simulink model "truckt_ROS_mpc_8dof_2020a"  (R2020a)
settings: Solver=FixedStepAuto  StartTime=0.0  StopTime=40  FixedStep=0.001  RelTol=1e-3
model workspace (MAT data in the model file):
  Logfile_Data_Object = robotics.ros.BagSelection
  Logfile_Data_Object.FilePath = 'D:\robotruck_school\robotruck_school\ws\2025-05-22-09-01-20-filter.bag'
  Logfile_Data_Object.StartTime = 1747875680.55
  Logfile_Data_Object.EndTime = 1747876785.76
  Logfile_Data_Object.NumMessages = 154547
  Logfile_Data_Object.AvailableTopics = table
  Logfile_Data_Object.AvailableTopics.data{1} = [32976; 55257; 12; 11050; 55252]
  Logfile_Data_Object.AvailableTopics.data{2} = categorical
  Logfile_Data_Object.AvailableTopics.data{2}.categoryNames = {'robominer_msgs/ControlCmd'; 'robominer_msgs/GlobalPlan'; 'robominer_msgs/LocalPlan'; 'robominer_msgs/LocalizationData'; 'robominer_msgs/VcuData'}
  Logfile_Data_Object.AvailableTopics.data{2}.codes = [1; 4; 2; 3; 5]
  Logfile_Data_Object.AvailableTopics.data{3}{1} = '  uint32 Seq
    |   Time Stamp
    |   char FrameId
    | robominer_msgs/DriveMode TargetDriveMode
    |   uint8 Mode
    |   uint8 MANU
    |   uint8 TELE
    |   uint8 AUTO
    |   uint8 JOYTELE
    | robominer_msgs/Gear TargetGear
    |   uint8 Gear
    |   uint8 P
    |   uint8 R
    |   uint8 N
    |   uint8 D
    |   uint8 ShiftError
    | robominer_msgs/GearData TargetGearData
    |   uint8 GearData
    |   uint8 DEFAULT
    |   uint8 N
    |   uint8 D1
    |   uint8 D2
    |   uint8 D3
    |   uint8 D4
    |   uint8 D5
    |   uint8 D6
    |   uint8 D7
    |   uint8 R
    |   uint8 R1
    |   uint8 R2
    |   uint8 DOWN
    |   uint8 UP
    |   uint8 ShiftError
    | double TargetThrottle
    | double TargetBrake
    | double TargetSteering
    | '
  Logfile_Data_Object.AvailableTopics.data{3}{2} = '  uint32 Seq
    |   Time Stamp
    |   char FrameId
    | logical IsValid
    | double Latitude
    | double Longitude
    | double Altitude
    | double X
    | double Y
    | double Z
    | double Speed
    | double Vx
    | double Vy
    | double Vz
    | double Ax
    | double Ay
    | double Az
    | double Roll
    | double Pitch
    | double Yaw
    | double Wx
    | double Wy
    | double Wz
    | uint8 Solnsvs
    | uint8 Solnsvs2
    | uint8 Age
    | uint8 GgaAge
    | robominer_msgs/LocalizationStatus RtkStatus
    |   uint8 Status
    |   uint8 RTKINIT
    |   uint8 APOSIT
    |   uint8 RTCMDIFF
    |   uint8 NOTUSED
    |   uint8 RTKFIX
    |   uint8 RTKFLO
    |   uint8 RTKOTHER
    |   uint8 DATATIMOUT
    | '
  Logfile_Data_Object.AvailableTopics.data{3}{3} = '  uint32 Seq
    |   Time Stamp
    |   char FrameId
    | robominer_msgs/Waypoints Waypoints
    |   robominer_msgs/Waypoint[] Points
    |     double X
    |     double Y
    |     double Z
    |     double Latitude
    |     double Longitude
    |     double Altitude
    |     double Yaw
    |     double Pitch
    |     double Speed
    |     double Steering
    |     double Fs
    |     double Kappa
    |     double SpeedLimit
    |     robominer_msgs/Gear Gear
    |       uint8 Gear
    |       uint8 P
    |       uint8 R
    |       uint8 N
    |       uint8 D
    |       uint8 ShiftError
    |     robominer_msgs/GearData GearData
    |       uint8 GearData
    |       uint8 DEFAULT
    |       uint8 N
    |       uint8 D1
    |       uint8 D2
    |       uint8 D3
    |       uint8 D4
    |       uint8 D5
    |       uint8 D6
    |       uint8 D7
    |       uint8 R
    |       uint8 R1
    |       uint8 R2
    |       uint8 DOWN
    |       uint8 UP
    |       uint8 ShiftError
    |     robominer_msgs/WaypointType WaypointType
    |       uint8 PointType
    |       uint8 NORMAL
    |       uint8 LOAD
    |       uint8 DUMP
    |       uint8 WAIT
    |       uint8 AVOID
    |       uint8 REGION
    |     uint32 Index
    | '
  Logfile_Data_Object.AvailableTopics.data{3}{4} = '  uint32 Seq
    |   Time Stamp
    |   char FrameId
    | robominer_msgs/TaskType TaskType
    |   uint32 Type
    |   uint32 NORMAL
    |   uint32 LOAD
    |   uint32 DUMP
    |   uint32 PARKING
    |   uint32 BATTERYSWAP
    |   uint32 OTHERTASKS
    | robominer_msgs/Waypoints Waypoints
    |   robominer_msgs/Waypoint[] Points
    |     double X
    |     double Y
    |     double Z
    |     double Latitude
    |     double Longitude
    |     double Altitude
    |     double Yaw
    |     double Pitch
    |     double Speed
    |     double Steering
    |     double Fs
    |     double Kappa
    |     double SpeedLimit
    |     robominer_msgs/Gear Gear
    |       uint8 Gear
    |       uint8 P
    |       uint8 R
    |       uint8 N
    |       uint8 D
    |       uint8 ShiftError
    |     robominer_msgs/GearData GearData
    |       uint8 GearData
    |       uint8 DEFAULT
    |       uint8 N
    |       uint8 D1
    |       uint8 D2
    |       uint8 D3
    |       uint8 D4
    |       uint8 D5
    |       uint8 D6
    |       uint8 D7
    |       uint8 R
    |       uint8 R1
    |       uint8 R2
    |       uint8 DOWN
    |       uint8 UP
    |       uint8 ShiftError
    |     robominer_msgs/WaypointType WaypointType
    |       uint8 PointType
    |       uint8 NORMAL
    |       uint8 LOAD
    |       uint8 DUMP
    |       uint8 WAIT
    |       uint8 AVOID
    |       uint8 REGION
    |     uint32 Index
    | robominer_msgs/PlanningStatus Status
    |   uint8 Status
    |   char Msg
    |   uint8 IDLE
    |   uint8 PAUSED
    |   uint8 RUNNING
    |   uint8 DONE
    |   uint8 FAIL
    |   uint8 PAUSING
    |   uint8 STOPING
    |   uint8 OBSTACLE
    |   uint8 CUSP
    |   uint8 PLANNING
    |   uint8 STOPYIELD
    |   uint8 PASSYIELD
    | int32 NearestPointIndex
    | double Fs
    | double Fd
    | double TotalFs
    | int32 ValidPointNum
    | double RefYaw
    | double YawDeviation
    | '
  Logfile_Data_Object.AvailableTopics.data{3}{5} : char (value not decoded)
  Logfile_Data_Object.AvailableTopics.ndims = 2
  Logfile_Data_Object.AvailableTopics.nrows = 5
  Logfile_Data_Object.AvailableTopics.rownames = {'/guardian/control_cmd'; '/localization/localization_data'; '/planner/global_path'; '/planner/local_path'; '/vcu/vcu_data'}
  Logfile_Data_Object.AvailableTopics.nvars = 3
  Logfile_Data_Object.AvailableTopics.varnames = {'NumMessages', 'MessageType', 'MessageDefinition'}
  Logfile_Data_Object.AvailableTopics.props.useVariableNamesOriginal = 0
  Logfile_Data_Object.AvailableTopics.props.useDimensionNamesOriginal = 0
  Logfile_Data_Object.AvailableTopics.props.CustomProps = struct()
  Logfile_Data_Object.AvailableTopics.props.VariableCustomProps = struct()
  Logfile_Data_Object.AvailableTopics.props.versionSavedFrom = 4
  Logfile_Data_Object.AvailableTopics.props.minCompatibleVersion = 1
  Logfile_Data_Object.AvailableTopics.props.incompatibilityMsg = ''
  Logfile_Data_Object.AvailableTopics.props.VersionSavedFrom = 4
  Logfile_Data_Object.AvailableTopics.props.Description = ''
  Logfile_Data_Object.AvailableTopics.props.VariableNamesOriginal = {}
  Logfile_Data_Object.AvailableTopics.props.DimensionNames = {'Row', 'Variables'}
  Logfile_Data_Object.AvailableTopics.props.DimensionNamesOriginal = {}
  Logfile_Data_Object.AvailableTopics.props.UserData = []
  Logfile_Data_Object.AvailableTopics.props.VariableDescriptions = {}
  Logfile_Data_Object.AvailableTopics.props.VariableUnits = {}
  Logfile_Data_Object.AvailableTopics.props.VariableContinuity = {}
  Logfile_Data_Object.MessageList = table
  Logfile_Data_Object.MessageList.data{1} = [1747875680.55 1747875680.56 1747875680.57 1747875680.59 1747875680.6 1747875680.61 1747875680.63 1747875680.63 1747875680.65 1747875680.66 1747875680.67 1747875680.69 ... (154547 elements, 154547x1)]
  Logfile_Data_Object.MessageList.data{2} = categorical
  Logfile_Data_Object.MessageList.data{2}.categoryNames = {'/guardian/control_cmd'; '/localization/localization_data'; '/planner/global_path'; '/planner/local_path'; '/vcu/vcu_data'}
  Logfile_Data_Object.MessageList.data{2}.codes = [2 1 2 2 1 2 2 1 2 1 2 2 ... (154547 elements, 154547x1)]
  Logfile_Data_Object.MessageList.data{3} = categorical
  Logfile_Data_Object.MessageList.data{3}.categoryNames = {'robominer_msgs/ControlCmd'; 'robominer_msgs/LocalizationData'; 'robominer_msgs/GlobalPlan'; 'robominer_msgs/LocalPlan'; 'robominer_msgs/VcuData'}
  Logfile_Data_Object.MessageList.data{3}.codes = [2 1 2 2 1 2 2 1 2 1 2 2 ... (154547 elements, 154547x1)]
  Logfile_Data_Object.MessageList.data{4} = [6172 8389 8478 8703 8928 9017 9242 9467 9556 9781 9870 10095 ... (154547 elements, 154547x1)]
  Logfile_Data_Object.MessageList.ndims = 2
  Logfile_Data_Object.MessageList.nrows = 154547
  Logfile_Data_Object.MessageList.nvars = 4
  Logfile_Data_Object.MessageList.varnames = {'Time', 'Topic', 'MessageType', 'FileOffset'}
  Logfile_Data_Object.MessageList.props.useVariableNamesOriginal = 0
  Logfile_Data_Object.MessageList.props.useDimensionNamesOriginal = 0
  Logfile_Data_Object.MessageList.props.CustomProps = struct()
  Logfile_Data_Object.MessageList.props.VariableCustomProps = struct()
  Logfile_Data_Object.MessageList.props.versionSavedFrom = 4
  Logfile_Data_Object.MessageList.props.minCompatibleVersion = 1
  Logfile_Data_Object.MessageList.props.incompatibilityMsg = ''
  Logfile_Data_Object.MessageList.props.VersionSavedFrom = 4
  Logfile_Data_Object.MessageList.props.Description = ''
  Logfile_Data_Object.MessageList.props.VariableNamesOriginal = {}
  Logfile_Data_Object.MessageList.props.DimensionNames = {'Row', 'Variables'}
  Logfile_Data_Object.MessageList.props.DimensionNamesOriginal = {}
  Logfile_Data_Object.MessageList.props.UserData = []
  Logfile_Data_Object.MessageList.props.VariableDescriptions = {}
  Logfile_Data_Object.MessageList.props.VariableUnits = {}
  Logfile_Data_Object.MessageList.props.VariableContinuity = {}
  Logfile_Data_Object.TopicTypeMap = containers.Map
  Logfile_Data_Object.TopicTypeMap.serialization.keys = {'/guardian/control_cmd', '/localization/localization_data', '/planner/global_path', '/planner/local_path', '/vcu/vcu_data'}
  Logfile_Data_Object.TopicTypeMap.serialization.values = {'robominer_msgs/ControlCmd', 'robominer_msgs/LocalizationData', 'robominer_msgs/GlobalPlan', 'robominer_msgs/LocalPlan', 'robominer_msgs/VcuData'}
  Logfile_Data_Object.TopicTypeMap.serialization.uniformity = 1
  Logfile_Data_Object.TopicTypeMap.serialization.keyType = 'char'
  Logfile_Data_Object.TopicTypeMap.serialization.valueType = 'char'
  Logfile_Data_Object.TopicDefinitionMap = containers.Map
  Logfile_Data_Object.TopicDefinitionMap.serialization.keys = {'/guardian/control_cmd', '/localization/localization_data', '/planner/global_path', '/planner/local_path', '/vcu/vcu_data'}
  Logfile_Data_Object.TopicDefinitionMap.serialization.values{1} = '  uint32 Seq
    |   Time Stamp
    |   char FrameId
    | robominer_msgs/DriveMode TargetDriveMode
    |   uint8 Mode
    |   uint8 MANU
    |   uint8 TELE
    |   uint8 AUTO
    |   uint8 JOYTELE
    | robominer_msgs/Gear TargetGear
    |   uint8 Gear
    |   uint8 P
    |   uint8 R
    |   uint8 N
    |   uint8 D
    |   uint8 ShiftError
    | robominer_msgs/GearData TargetGearData
    |   uint8 GearData
    |   uint8 DEFAULT
    |   uint8 N
    |   uint8 D1
    |   uint8 D2
    |   uint8 D3
    |   uint8 D4
    |   uint8 D5
    |   uint8 D6
    |   uint8 D7
    |   uint8 R
    |   uint8 R1
    |   uint8 R2
    |   uint8 DOWN
    |   uint8 UP
    |   uint8 ShiftError
    | double TargetThrottle
    | double TargetBrake
    | double TargetSteering
    | '
  Logfile_Data_Object.TopicDefinitionMap.serialization.values{2} = '  uint32 Seq
    |   Time Stamp
    |   char FrameId
    | logical IsValid
    | double Latitude
    | double Longitude
    | double Altitude
    | double X
    | double Y
    | double Z
    | double Speed
    | double Vx
    | double Vy
    | double Vz
    | double Ax
    | double Ay
    | double Az
    | double Roll
    | double Pitch
    | double Yaw
    | double Wx
    | double Wy
    | double Wz
    | uint8 Solnsvs
    | uint8 Solnsvs2
    | uint8 Age
    | uint8 GgaAge
    | robominer_msgs/LocalizationStatus RtkStatus
    |   uint8 Status
    |   uint8 RTKINIT
    |   uint8 APOSIT
    |   uint8 RTCMDIFF
    |   uint8 NOTUSED
    |   uint8 RTKFIX
    |   uint8 RTKFLO
    |   uint8 RTKOTHER
    |   uint8 DATATIMOUT
    | '
  Logfile_Data_Object.TopicDefinitionMap.serialization.values{3} = '  uint32 Seq
    |   Time Stamp
    |   char FrameId
    | robominer_msgs/Waypoints Waypoints
    |   robominer_msgs/Waypoint[] Points
    |     double X
    |     double Y
    |     double Z
    |     double Latitude
    |     double Longitude
    |     double Altitude
    |     double Yaw
    |     double Pitch
    |     double Speed
    |     double Steering
    |     double Fs
    |     double Kappa
    |     double SpeedLimit
    |     robominer_msgs/Gear Gear
    |       uint8 Gear
    |       uint8 P
    |       uint8 R
    |       uint8 N
    |       uint8 D
    |       uint8 ShiftError
    |     robominer_msgs/GearData GearData
    |       uint8 GearData
    |       uint8 DEFAULT
    |       uint8 N
    |       uint8 D1
    |       uint8 D2
    |       uint8 D3
    |       uint8 D4
    |       uint8 D5
    |       uint8 D6
    |       uint8 D7
    |       uint8 R
    |       uint8 R1
    |       uint8 R2
    |       uint8 DOWN
    |       uint8 UP
    |       uint8 ShiftError
    |     robominer_msgs/WaypointType WaypointType
    |       uint8 PointType
    |       uint8 NORMAL
    |       uint8 LOAD
    |       uint8 DUMP
    |       uint8 WAIT
    |       uint8 AVOID
    |       uint8 REGION
    |     uint32 Index
    | '
  Logfile_Data_Object.TopicDefinitionMap.serialization.values{4} = '  uint32 Seq
    |   Time Stamp
    |   char FrameId
    | robominer_msgs/TaskType TaskType
    |   uint32 Type
    |   uint32 NORMAL
    |   uint32 LOAD
    |   uint32 DUMP
    |   uint32 PARKING
    |   uint32 BATTERYSWAP
    |   uint32 OTHERTASKS
    | robominer_msgs/Waypoints Waypoints
    |   robominer_msgs/Waypoint[] Points
    |     double X
    |     double Y
    |     double Z
    |     double Latitude
    |     double Longitude
    |     double Altitude
    |     double Yaw
    |     double Pitch
    |     double Speed
    |     double Steering
    |     double Fs
    |     double Kappa
    |     double SpeedLimit
    |     robominer_msgs/Gear Gear
    |       uint8 Gear
    |       uint8 P
    |       uint8 R
    |       uint8 N
    |       uint8 D
    |       uint8 ShiftError
    |     robominer_msgs/GearData GearData
    |       uint8 GearData
    |       uint8 DEFAULT
    |       uint8 N
    |       uint8 D1
    |       uint8 D2
    |       uint8 D3
    |       uint8 D4
    |       uint8 D5
    |       uint8 D6
    |       uint8 D7
    |       uint8 R
    |       uint8 R1
    |       uint8 R2
    |       uint8 DOWN
    |       uint8 UP
    |       uint8 ShiftError
    |     robominer_msgs/WaypointType WaypointType
    |       uint8 PointType
    |       uint8 NORMAL
    |       uint8 LOAD
    |       uint8 DUMP
    |       uint8 WAIT
    |       uint8 AVOID
    |       uint8 REGION
    |     uint32 Index
    | robominer_msgs/PlanningStatus Status
    |   uint8 Status
    |   char Msg
    |   uint8 IDLE
    |   uint8 PAUSED
    |   uint8 RUNNING
    |   uint8 DONE
    |   uint8 FAIL
    |   uint8 PAUSING
    |   uint8 STOPING
    |   uint8 OBSTACLE
    |   uint8 CUSP
    |   uint8 PLANNING
    |   uint8 STOPYIELD
    |   uint8 PASSYIELD
    | int32 NearestPointIndex
    | double Fs
    | double Fd
    | double TotalFs
    | int32 ValidPointNum
    | double RefYaw
    | double YawDeviation
    | '
  Logfile_Data_Object.TopicDefinitionMap.serialization.values{5} : char (value not decoded)
  Logfile_Data_Object.TopicDefinitionMap.serialization.uniformity = 1
  Logfile_Data_Object.TopicDefinitionMap.serialization.keyType = 'char'
  Logfile_Data_Object.TopicDefinitionMap.serialization.valueType = 'char'
  Logfile_Data_Object.Parser = robotics.ros.internal.tf.TransformationTreeParser
  Logfile_Path = 'D:\robotruck_school\robotruck_school\ws\2025-05-22-09-01-20-filter.bag'
  Logfile_Playback_Duration = nan
  Logfile_Playback_Offset = nan
undefined symbols (not defined in the file): Ax, Ay, Header, SteeringAngle, Vx, Vy, WheelSpeedFl, WheelSpeedFr, X, Y, Yaw
libraries: neural x31, robotlib x5, simulink x2, Solver_SF x1
(part 1 of 2)
settings Model: Creator=pc  LastModifiedBy=lenovo
settings DebuggingCC: UnconnectedInputMsg=none  UnconnectedOutputMsg=none  UnconnectedLineMsg=none
settings ModelReferenceCC: EnableRefExpFcnMdlSchedulingChecks=off
settings RTWCC: Description=Generic Real-Time Target

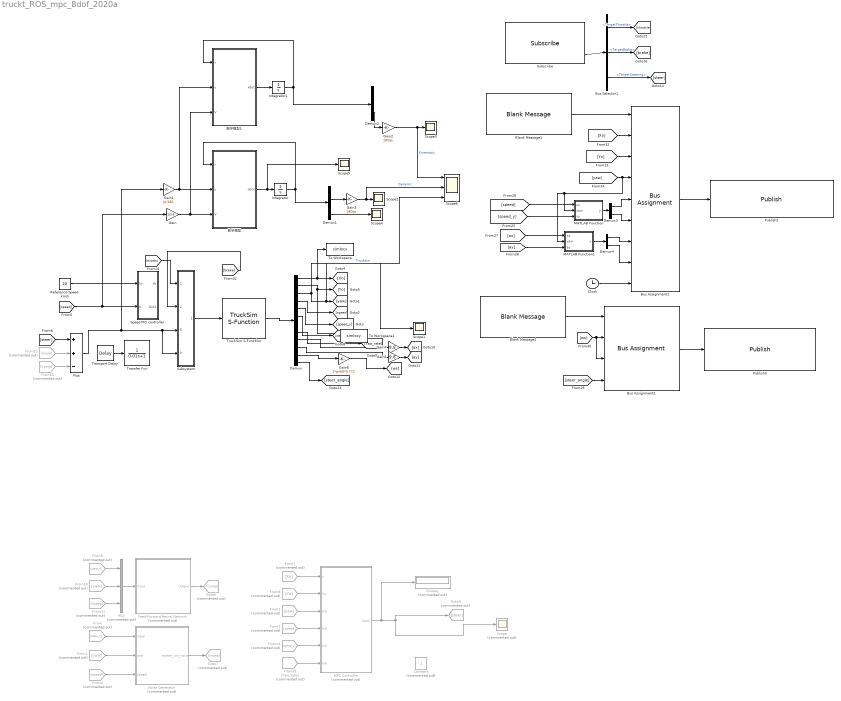
== system truckt_ROS_mpc_8dof_2020a ==
  Blank Message1 : robotlib/Blank Message  messageClass=Message  entityType=robominer_msgs/LocalizationData  messageType=robominer_msgs/LocalizationData  SampleTime=inf
  Blank Message2 : robotlib/Blank Message  messageClass=Message  entityType=robominer_msgs/VcuData  messageType=robominer_msgs/VcuData  SampleTime=inf
  Bus Assignment1 : BusAssignment  AssignedSignals=X,Y,Yaw,Vx,Vy,Ax,Ay,Header.Stamp.Sec
  Bus Assignment2 : BusAssignment  AssignedSignals=WheelSpeedFl,WheelSpeedFr,SteeringAngle
  Bus Selector1 : BusSelector  OutputSignals=TargetThrottle,TargetBrake,TargetSteering
  Clock : Clock
  Constant : Constant  Commented=on
  Demux : Demux  Outputs=12
  Demux1 : Demux
  Demux2 : Demux  Outputs=2
  Demux3 : Demux  Outputs=2
  Demux4 : Demux  Outputs=2
  Display : Display  Commented=on
  Feed-Forward Neural Network : Subsystem  Commented=on
      mask help: Feed-Forward Neural Network
      mask Display: e = 0.06;c1 = [120 150 230]/255;c2 = ([120 150 230]+0)/383;c3 = ([120 150 230]+128)/383;patch([0 1 1 0],[0 0 1 1],c1);patch([0 1 1 1-e 1-e 0+e],[0 0 1 1-e 0+e 0+e],c2);patch([0 0 1 1-e 0+e 0+e],[0 1 1 1-e 1-e 0+e],c3);plot([0 1 1 0 0],[0 0 1 1 0]);fprintf('NNET');port_label('input',1,' Input');port_label('output',1,'Output ');
  From : From  Commented=on  GotoTag=steer_fl
  From1 : From  Commented=on  GotoTag=yaw
  From10 : From  Commented=on  GotoTag=yaw
  From11 : From  Commented=on  GotoTag=speed
  From12 : From  Commented=on  GotoTag=noise
  From13 : From  Commented=on  GotoTag=comp
  From14 : From  Commented=on  GotoTag=speed_y
  From15 : From  Commented=on  GotoTag=Yaw_rate
  From2 : From  Commented=on  GotoTag=yaw
  From3 : From  Commented=on  GotoTag=speed
  From4 : From  Commented=on  GotoTag=speed
  From7 : From  Commented=on  GotoTag=Xo
  From8 : From  Commented=on  GotoTag=Yo
  From9 : From  Commented=on  GotoTag=steer_fl
  Gain : Gain  Gain=1/3.6
  Gain1 : Gain  Gain=pi/180
  Gain2 : Gain  Gain=180/pi
  Gain3 : Gain  Gain=180/pi
  Gain4 : Gain  Gain=9.8
  Gain5 : Gain  Gain=9.8
  Gain6 : Gain  Gain=2*pi/60*0.772
  Goto3 : Goto  Commented=on  GotoTag=steer
  Goto6 : Goto  Commented=on  GotoTag=comp
  Goto7 : Goto  Commented=on  GotoTag=noise
  Integrator : Integrator  InitialCondition=[0;0;0;0]
  Integrator1 : Integrator  InitialCondition=[0;0]
  MATLAB Function : MATLAB Function  TreatAsAtomicUnit=on
  MATLAB Function1 : MATLAB Function  TreatAsAtomicUnit=on
  MPC Controller : Subsystem  Commented=on
  Mux : Mux  Commented=on  Inputs=3
  Noise Generator : MATLAB Function  Commented=on  TreatAsAtomicUnit=on
  Plus : Sum  Inputs=++-
  Publish2 : robotlib/Publish  topicSource=Specify your own  topic=/localization/localization_data  messageType=robominer_msgs/LocalizationData  messageQueueLength=1
  Publish3 : robotlib/Publish  topicSource=Specify your own  topic=/vcu/vcu_data  messageType=robominer_msgs/VcuData  messageQueueLength=1
  Reference Speed km/h : Constant  Value=20
  Scope : Scope  Commented=on
  Scope{1..5} (5 alike) : Scope
  Scope6 : Scope  NumInputPorts=3
  Speed PID controller : Subsystem
  Subscribe : robotlib/Subscribe  topicSource=Specify your own  topic=/guardian/control_cmd  messageType=robominer_msgs/ControlCmd  sampleTime=-1  messageQueueLength=1
  Subsystem : Subsystem
  To Workspace : ToWorkspace  VariableName=simlocx  SaveFormat=Timeseries  SampleTime=-1
  To Workspace1 : ToWorkspace  VariableName=simlocy  SaveFormat=Timeseries  SampleTime=-1
  Transfer Fcn : TransferFcn  Denominator=[0.01 1]
  Transport Delay : TransportDelay  DelayTime=0.2
  TruckSim S-Function : Solver_SF/TruckSim S-Function  Priority=1  SIMFILE=simfile.sim
      settings: SourceProductName=CarSim S-Function
  数学模型 : MATLAB Function  TreatAsAtomicUnit=on
  数学模型1 : MATLAB Function  TreatAsAtomicUnit=on
  wires:
  TruckSim S-Function/1 -> Demux/1
  Demux/4 -> [speed]
  Subsystem/1(Out1) -> TruckSim S-Function/1
  Demux/2 -> To Workspace1/1, [Yo]
  Demux/1 -> To Workspace/1, [Xo]
  Reference Speed km/h/1 -> Speed PID controller/1(Vr)
  Transport Delay/1 -> Transfer Fcn/1
  Mux/1 -> Feed-Forward Neural Network/1(Input)
  Demux/5 -> [speed_y]
  From/1 -> Noise Generator/1(steer)
  Demux/3 -> Scope6/3, [yaw], Scope1/1  "Trucksim"
  From1/1 -> Noise Generator/2(yaw)
  From4/1 -> Noise Generator/3(speed)
  [speed] -> Gain/1, Speed PID controller/2(V)
  From7/1 -> MPC Controller/1(x)
  From8/1 -> MPC Controller/2(Yo)
  From2/1 -> MPC Controller/3(In3)
  From3/1 -> MPC Controller/4(In4)
  MPC Controller/1(Out1) -> Display/1, Scope/1, Goto3/1
  From10/1 -> Mux/2
  From11/1 -> Mux/3
  From9/1 -> Mux/1
  Feed-Forward Neural Network/1(Output) -> Goto6/1
  Noise Generator/1(esteer_sin_noise) -> Goto7/1
  From12/1 -> Plus/2
  From13/1 -> Plus/3
  Plus/1 -> Gain1/1, Subsystem/4(fr), Subsystem/3(fl)
  Demux/6 -> [steer_fl]
  From14/1 -> MPC Controller/5(In5)
  Demux/8 -> [Yaw_rate]
  From15/1 -> MPC Controller/6(In6)
  [steer] -> Plus/1
  数学模型/1(dotx) -> Scope5/1, Integrator/1
  Integrator/1 -> Demux1/1, 数学模型/1(x)
  Demux1/2 -> Gain3/1
  Gain/1 -> 数学模型1/3(V), 数学模型/3(V)
  Gain1/1 -> 数学模型1/2(u), 数学模型/2(u)
  数学模型1/1(xdot) -> Integrator1/1
  Integrator1/1 -> 数学模型1/1(x), Demux2/1
  Demux2/2 -> Gain2/1
  Gain2/1 -> Scope6/1, Scope3/1  "Kinematic"
  Demux1/4 -> Scope4/1
  Gain3/1 -> Scope6/2, Scope2/1  "Dynamic"
  Bus Assignment1/1 -> Publish2/1
  Blank Message1/1 -> Bus Assignment1/1
  Subscribe/2 -> Bus Selector1/1
  [Xo] -> Bus Assignment1/2
  [Yo] -> Bus Assignment1/3
  [yaw] -> Bus Assignment1/4, MATLAB Function/2(yaw), MATLAB Function1/2(yaw)
  Clock/1 -> Bus Assignment1/9
  Blank Message2/1 -> Bus Assignment2/1
  Bus Assignment2/1 -> Publish3/1
  [speed] -> MATLAB Function/1(vx)
  [speed_y] -> MATLAB Function/3(vy)
  MATLAB Function/1(y) -> Demux3/1
  Demux3/1 -> Bus Assignment1/5
  Demux3/2 -> Bus Assignment1/6
  Demux/9 -> Gain4/1
  Gain4/1 -> [ax]
  Demux/10 -> Gain5/1
  Gain5/1 -> [ay]
  [ax] -> MATLAB Function1/1(ax)
  [ay] -> MATLAB Function1/3(ay)
  MATLAB Function1/1(y) -> Demux4/1
  Demux4/2 -> Bus Assignment1/8
  Demux4/1 -> Bus Assignment1/7
  Demux/11 -> Gain6/1
  Gain6/1 -> [ws]
  Demux/12 -> [steer_angle]
  [ws] -> Bus Assignment2/3, Bus Assignment2/2
  [steer_angle] -> Bus Assignment2/4
  Bus Selector1/3 -> [steer]  "<TargetSteering>"
  Bus Selector1/1 -> [throttle]  "<TargetThrottle>"
  Bus Selector1/2 -> [brake]  "<TargetBrake>"
  [throttle] -> Subsystem/1(In3)
  [brake] -> Subsystem/2(In4)

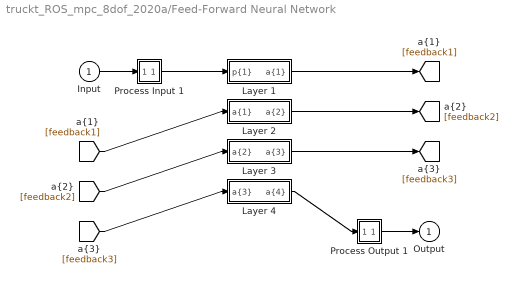
== system truckt_ROS_mpc_8dof_2020a/Feed-Forward Neural Network ==
  Input : Inport  PortDimensions=3  SampleTime=0.0005
      mask Display: e = 0.06;c1 = [120 230 180]/255;c2 = ([120 230 180]+0)/(256+128);c3 = ([120 230 180]+128)/(256+128);patch([0 1 1 0],[0 0 1 1],c1);patch([0 1 1 1-e 1-e 0+e],[0 0 1 1-e 0+e 0+e],c2);patch([0 0 1 1-e 0+e 0+e],[0 1 1 1-e 1-e 0+e],c3);plot([0 1 1 0 0],[0 0 1 1 0]);
  Layer 1 : Subsystem
      mask Display: e = 0.06;c1 = [120 150 230]/255;c2 = ([120 150 230]+0)/383;c3 = ([120 150 230]+128)/383;patch([0 1 1 0],[0 0 1 1],c1);patch([0 1 1 1-e 1-e 0+e],[0 0 1 1-e 0+e 0+e],c2);patch([0 0 1 1-e 0+e 0+e],[0 1 1 1-e 1-e 0+e],c3);plot([0 1 1 0 0],[0 0 1 1 0]);
  Layer 2 : Subsystem
      mask Display: e = 0.06;c1 = [120 150 230]/255;c2 = ([120 150 230]+0)/383;c3 = ([120 150 230]+128)/383;patch([0 1 1 0],[0 0 1 1],c1);patch([0 1 1 1-e 1-e 0+e],[0 0 1 1-e 0+e 0+e],c2);patch([0 0 1 1-e 0+e 0+e],[0 1 1 1-e 1-e 0+e],c3);plot([0 1 1 0 0],[0 0 1 1 0]);
  Layer 3 : Subsystem
      mask Display: e = 0.06;c1 = [120 150 230]/255;c2 = ([120 150 230]+0)/383;c3 = ([120 150 230]+128)/383;patch([0 1 1 0],[0 0 1 1],c1);patch([0 1 1 1-e 1-e 0+e],[0 0 1 1-e 0+e 0+e],c2);patch([0 0 1 1-e 0+e 0+e],[0 1 1 1-e 1-e 0+e],c3);plot([0 1 1 0 0],[0 0 1 1 0]);
  Layer 4 : Subsystem
      mask Display: e = 0.06;c1 = [120 150 230]/255;c2 = ([120 150 230]+0)/383;c3 = ([120 150 230]+128)/383;patch([0 1 1 0],[0 0 1 1],c1);patch([0 1 1 1-e 1-e 0+e],[0 0 1 1-e 0+e 0+e],c2);patch([0 0 1 1-e 0+e 0+e],[0 1 1 1-e 1-e 0+e],c3);plot([0 1 1 0 0],[0 0 1 1 0]);
  Process Input 1 : Subsystem
      mask Display: e = 0.06;c1 = [120 150 230]/255;c2 = ([120 150 230]+0)/383;c3 = ([120 150 230]+128)/383;patch([0 1 1 0],[0 0 1 1],c1);patch([0 1 1 1-e 1-e 0+e],[0 0 1 1-e 0+e 0+e],c2);patch([0 0 1 1-e 0+e 0+e],[0 1 1 1-e 1-e 0+e],c3);plot([0 1 1 0 0],[0 0 1 1 0]);
  Process Output 1 : Subsystem
      mask Display: e = 0.06;c1 = [120 150 230]/255;c2 = ([120 150 230]+0)/383;c3 = ([120 150 230]+128)/383;patch([0 1 1 0],[0 0 1 1],c1);patch([0 1 1 1-e 1-e 0+e],[0 0 1 1-e 0+e 0+e],c2);patch([0 0 1 1-e 0+e 0+e],[0 1 1 1-e 1-e 0+e],c3);plot([0 1 1 0 0],[0 0 1 1 0]);
  Output : Outport  InitialOutput=0
      mask Display: e = 0.06;c1 = [120 230 180]/255;c2 = ([120 230 180]+0)/(256+128);c3 = ([120 230 180]+128)/(256+128);patch([0 1 1 0],[0 0 1 1],c1);patch([0 1 1 1-e 1-e 0+e],[0 0 1 1-e 0+e 0+e],c2);patch([0 0 1 1-e 0+e 0+e],[0 1 1 1-e 1-e 0+e],c3);plot([0 1 1 0 0],[0 0 1 1 0]);
  wires:
  Input/1 -> Process Input 1/1(x)
  Process Output 1/1(y) -> Output/1
  Process Input 1/1(p) -> Layer 1/1("p{1}")
  Layer 1/1("a{1}") -> [feedback1]
  [feedback1] -> Layer 2/1("a{1} ")
  Layer 2/1("a{2}") -> [feedback2]
  [feedback2] -> Layer 3/1("a{2} ")
  Layer 3/1("a{3}") -> [feedback3]
  [feedback3] -> Layer 4/1("a{3} ")
  Layer 4/1("a{4}") -> Process Output 1/1(a)

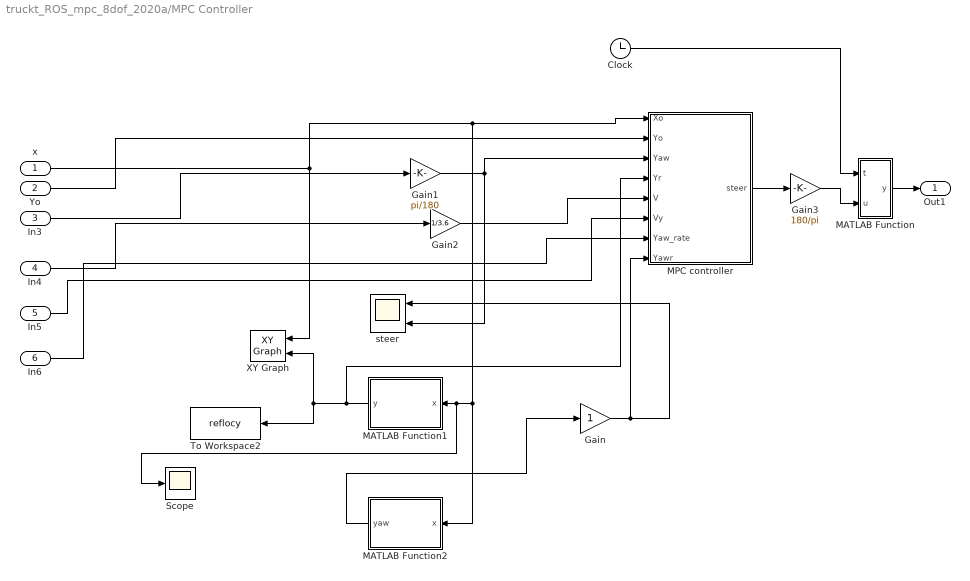
== system truckt_ROS_mpc_8dof_2020a/MPC Controller ==
  x : Inport
  Yo : Inport  Port=2
  In3 : Inport  Port=3
  In4 : Inport  Port=4
  In5 : Inport  Port=5
  In6 : Inport  Port=6
  Clock : Clock
  Gain : Gain
  Gain1 : Gain  Gain=pi/180
  Gain2 : Gain  Gain=1/3.6
  Gain3 : Gain  Gain=180/pi
  MATLAB Function : MATLAB Function  TreatAsAtomicUnit=on
  MATLAB Function1 : MATLAB Function  TreatAsAtomicUnit=on
  MATLAB Function2 : MATLAB Function  TreatAsAtomicUnit=on
  MPC controller : MATLAB Function  TreatAsAtomicUnit=on
  Scope : Scope
  To Workspace2 : ToWorkspace  VariableName=reflocy  SaveFormat=Timeseries  SampleTime=-1
  XY Graph : simulink/Sinks/XY Graph  xmin=-1  xmax=1  ymin=-1  ymax=1  st=-1
  steer : Scope  NumInputPorts=2
  Out1 : Outport
  wires:
  MATLAB Function2/1(yaw) -> Gain/1
  Gain1/1 -> steer/2, MPC controller/3(Yaw)
  Gain/1 -> steer/1, MPC controller/8(Yawr)
  Gain2/1 -> MPC controller/5(V)
  In4/1 -> Gain2/1
  In3/1 -> Gain1/1
  MATLAB Function1/1(y) -> To Workspace2/1, XY Graph/2, MPC controller/4(Yr)
  MPC controller/1(steer) -> Gain3/1
  x/1 -> Scope/1, MATLAB Function1/1(x), MATLAB Function2/1(x), MPC controller/1(Xo), XY Graph/1
  Gain3/1 -> MATLAB Function/2(u)
  Yo/1 -> MPC controller/2(Yo)
  In5/1 -> MPC controller/6(Vy)
  In6/1 -> MPC controller/7(Yaw_rate)
  MATLAB Function/1(y) -> Out1/1
  Clock/1 -> MATLAB Function/1(t)

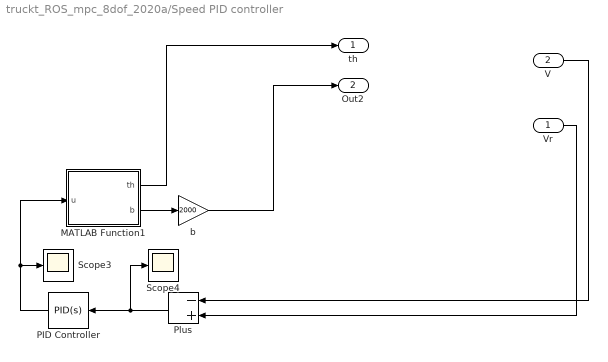
== system truckt_ROS_mpc_8dof_2020a/Speed PID controller ==
  Vr : Inport
  V : Inport  Port=2
  MATLAB Function1 : MATLAB Function  TreatAsAtomicUnit=on
  PID Controller : simulink/Continuous/PID Controller  Controller=PID  Form=Parallel  TimeDomain=Continuous-time  UseExternalTs=off  SampleTime=-1  IntegratorMethod=Forward Euler  FilterMethod=Forward Euler  ControllerParametersSource=internal  P=5  I=1  D=1  UseFilter=on  N=100  TunerSelectOption=Transfer Function Based (PID Tuner App)  InitialConditionSource=internal  InitialConditionForIntegrator=0  InitialConditionForFilter=0  DifferentiatorICPrevScaledInput=0  ExternalReset=none  TrackingMode=off  Kt=1  LimitOutput=off  UpperSaturationLimit=inf  LowerSaturationLimit=-inf  LinearizeAsGain=on  AntiWindupMode=none  Kb=1  POutMin=[]  POutMax=[]  IOutMin=[]  IOutMax=[]  DOutMin=[]  DOutMax=[]  NOutMin=[]  NOutMax=[]  SumOutMin=[]  SumOutMax=[]  SaturationOutMin=[]  SaturationOutMax=[]  PParamMin=[]  PParamMax=[]  IParamMin=[]  IParamMax=[]  DParamMin=[]  DParamMax=[]  NParamMin=[]  NParamMax=[]  KbParamMin=[]  KbParamMax=[]  KtParamMin=[]  KtParamMax=[]  KbOutMin=[]  KbOutMax=[]  KtOutMin=[]  KtOutMax=[]  IntegratorOutMin=[]  IntegratorOutMax=[]  FilterOutMin=[]  FilterOutMax=[]  SumI1OutMin=[]  SumI1OutMax=[]  SumI2OutMin=[]  SumI2OutMax=[]  SumI3OutMin=[]  SumI3OutMax=[]  SumI4OutMin=[]  SumI4OutMax=[]  SumDOutMin=[]  SumDOutMax=[]  DifferentiatorOutMin=[]  DifferentiatorOutMax=[]  FilterDiffOutCoefMin=[]  FilterDiffOutCoefMax=[]  ReciprocalOutMin=[]  ReciprocalOutMax=[]  SumDenOutMin=[]  SumDenOutMax=[]  SumNumOutMin=[]  SumNumOutMax=[]  DivideOutMin=[]  DivideOutMax=[]  UdiffTsProdOutMin=[]  UdiffTsProdOutMax=[]  NTsProdOutMin=[]  NTsProdOutMax=[]  UintegralTsProdOutMin=[]  UintegralTsProdOutMax=[]  UngainTsProdOutMin=[]  UngainTsProdOutMax=[]  IntegratorContinuousStateAttributes=''  IntegratorStateMustResolveToSignalObject=off  IntegratorRTWStateStorageClass=Auto  FilterContinuousStateAttributes=''  FilterStateMustResolveToSignalObject=off  FilterRTWStateStorageClass=Auto  ParallelPVariant=InternalParameters  IdealPVariant=Disabled  IVariant=InternalParameters  DVariant=InternalParameters  IntegratorVariant=Continuous  SatVariant=Disabled  AWVariant=Passthrough  PCopyVariant=Disabled  TRVariant=Disabled  FdbkBlocksVariant=Forward  IdealPFdbkVariant=Disabled  SatFdbkVariant=Disabled  DerivativeFilterVariant=ContFilter  NVariant=InternalParameters  NCopyVariant=Disabled  FilterICVariant=InternalICsFilter  IntegratorICVariant=InternalICs  ExternalResetVariant=Disabled  TRSumVariant=Passthrough  SumFdbkVariant=Disabled  SumVariant=Sum_PID  TsampFilterVariant=InternalTs  TsampNgainVariant=Passthrough  TsampIntegralVariant=Passthrough
  Plus : Sum  Inputs=-+
  Scope3 : Scope
  Scope4 : Scope
  b : Gain  Gain=2000
  th : Outport
  Out2 : Outport  Port=2
  wires:
  MATLAB Function1/1(th) -> th/1
  MATLAB Function1/2(b) -> b/1
  Plus/1 -> PID Controller/1, Scope4/1
  b/1 -> Out2/1
  Vr/1 -> Plus/2
  V/1 -> Plus/1
  PID Controller/1 -> MATLAB Function1/1(u), Scope3/1

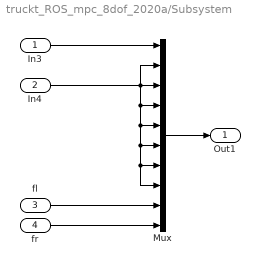
== system truckt_ROS_mpc_8dof_2020a/Subsystem ==
  In3 : Inport
  In4 : Inport  Port=2
  fl : Inport  Port=3
  fr : Inport  Port=4
  Mux : Mux  Inputs=10
  Out1 : Outport
  wires:
  Mux/1 -> Out1/1
  In4/1 -> Mux/8, Mux/7, Mux/6, Mux/5, Mux/4, Mux/3, Mux/2
  In3/1 -> Mux/1
  fl/1 -> Mux/9
  fr/1 -> Mux/10

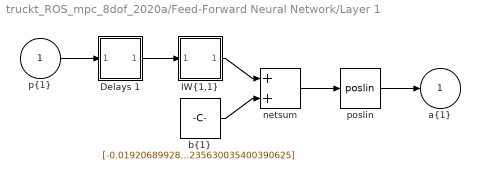
== system truckt_ROS_mpc_8dof_2020a/Feed-Forward Neural Network/Layer 1 ==
  "p{1}" : Inport  PortDimensions=3  SampleTime=0.0005
      mask Display: e = 0.06;c1 = [120 230 180]/255;c2 = ([120 230 180]+0)/(256+128);c3 = ([120 230 180]+128)/(256+128);patch([0 1 1 0],[0 0 1 1],c1);patch([0 1 1 1-e 1-e 0+e],[0 0 1 1-e 0+e 0+e],c2);patch([0 0 1 1-e 0+e 0+e],[0 1 1 1-e 1-e 0+e],c3);plot([0 1 1 0 0],[0 0 1 1 0]);
  Delays 1 : Subsystem
      mask Display: e = 0.06;c1 = [120 150 230]/255;c2 = ([120 150 230]+0)/383;c3 = ([120 150 230]+128)/383;patch([0 1 1 0],[0 0 1 1],c1);patch([0 1 1 1-e 1-e 0+e],[0 0 1 1-e 0+e 0+e],c2);patch([0 0 1 1-e 0+e 0+e],[0 1 1 1-e 1-e 0+e],c3);plot([0 1 1 0 0],[0 0 1 1 0]);disp('0');
  "IW{1,1}" : Subsystem
      mask Display: e = 0.06;c1 = [120 150 230]/255;c2 = ([120 150 230]+0)/383;c3 = ([120 150 230]+128)/383;patch([0 1 1 0],[0 0 1 1],c1);patch([0 1 1 1-e 1-e 0+e],[0 0 1 1-e 0+e 0+e],c2);patch([0 0 1 1-e 0+e 0+e],[0 1 1 1-e 1-e 0+e],c3);plot([0 1 1 0 0],[0 0 1 1 0]);disp('W');
  "b{1}" : Constant  Value=[-0.0192068992804849403288613984841504134237766265869140625;0.89827192612352446676737827147007919847965240478515625;0.141640567856664068013827773029333911836147308349609375;-0.358637837925329938659757544883177615702152252197265625;-0.5661933112486650099270946157048456370830535888671875;0.64533946781671824854953456451767124235630035400390625]
      mask Display: e = 0.06;c1 = [120 150 230]/255;c2 = ([120 150 230]+0)/383;c3 = ([120 150 230]+128)/383;patch([0 1 1 0],[0 0 1 1],c1);patch([0 1 1 1-e 1-e 0+e],[0 0 1 1-e 0+e 0+e],c2);patch([0 0 1 1-e 0+e 0+e],[0 1 1 1-e 1-e 0+e],c3);plot([0 1 1 0 0],[0 0 1 1 0]);disp('b');
  netsum : Sum  Inputs=2  InputSameDT=on  SaturateOnIntegerOverflow=on  OutDataTypeStr=Inherit: Same as first input
      mask Display: e = 0.06;c1 = [120 150 230]/255;c2 = ([120 150 230]+0)/383;c3 = ([120 150 230]+128)/383;patch([0 1 1 0],[0 0 1 1],c1);patch([0 1 1 1-e 1-e 0+e],[0 0 1 1-e 0+e 0+e],c2);patch([0 0 1 1-e 0+e 0+e],[0 1 1 1-e 1-e 0+e],c3);plot([0 1 1 0 0],[0 0 1 1 0]);disp('+');
  poslin : neural/Transfer Functions/poslin
      settings: SourceProductBaseCode=NN
  "a{1}" : Outport  InitialOutput=[0;0;0;0;0;0]
      mask Display: e = 0.06;c1 = [120 230 180]/255;c2 = ([120 230 180]+0)/(256+128);c3 = ([120 230 180]+128)/(256+128);patch([0 1 1 0],[0 0 1 1],c1);patch([0 1 1 1-e 1-e 0+e],[0 0 1 1-e 0+e 0+e],c2);patch([0 0 1 1-e 0+e 0+e],[0 1 1 1-e 1-e 0+e],c3);plot([0 1 1 0 0],[0 0 1 1 0]);
  wires:
  "p{1}"/1 -> Delays 1/1("p{1}")
  Delays 1/1("pd{1,1}") -> "IW{1,1}"/1("pd{1,1}")
  "IW{1,1}"/1("iz{1,1}") -> netsum/1
  "b{1}"/1 -> netsum/2
  netsum/1 -> poslin/1
  poslin/1 -> "a{1}"/1

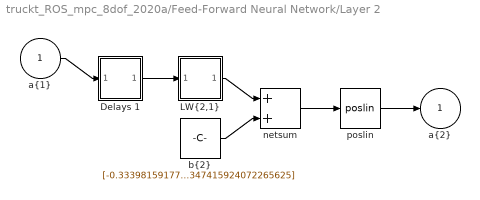
== system truckt_ROS_mpc_8dof_2020a/Feed-Forward Neural Network/Layer 2 ==
  "a{1} " : Inport  PortDimensions=6  SampleTime=0.0005
      mask Display: e = 0.06;c1 = [120 230 180]/255;c2 = ([120 230 180]+0)/(256+128);c3 = ([120 230 180]+128)/(256+128);patch([0 1 1 0],[0 0 1 1],c1);patch([0 1 1 1-e 1-e 0+e],[0 0 1 1-e 0+e 0+e],c2);patch([0 0 1 1-e 0+e 0+e],[0 1 1 1-e 1-e 0+e],c3);plot([0 1 1 0 0],[0 0 1 1 0]);
  Delays 1 : Subsystem
      mask Display: e = 0.06;c1 = [120 150 230]/255;c2 = ([120 150 230]+0)/383;c3 = ([120 150 230]+128)/383;patch([0 1 1 0],[0 0 1 1],c1);patch([0 1 1 1-e 1-e 0+e],[0 0 1 1-e 0+e 0+e],c2);patch([0 0 1 1-e 0+e 0+e],[0 1 1 1-e 1-e 0+e],c3);plot([0 1 1 0 0],[0 0 1 1 0]);disp('0');
  "LW{2,1}" : Subsystem
      mask Display: e = 0.06;c1 = [120 150 230]/255;c2 = ([120 150 230]+0)/383;c3 = ([120 150 230]+128)/383;patch([0 1 1 0],[0 0 1 1],c1);patch([0 1 1 1-e 1-e 0+e],[0 0 1 1-e 0+e 0+e],c2);patch([0 0 1 1-e 0+e 0+e],[0 1 1 1-e 1-e 0+e],c3);plot([0 1 1 0 0],[0 0 1 1 0]);disp('W');
  "b{2}" : Constant  Value=[-0.333981591773017394420008940869593061506748199462890625;0.78211470382805980960938541102223098278045654296875;0.79995506424217988072911111885332502424716949462890625;-0.2460003254337694844622319578775204718112945556640625;-0.8654396309132881270897996728308498859405517578125;-0.5946510837343403910182360050384886562824249267578125;0.044554086099510982477145404345719725824892520904541015625;-0.178063550368801892798131802919670008122920989990234375;-0.44061723010858722116012131664319895207881927490234375;-0.395553500913042810349651290380279533565044403076171875;-0.4019893215360192950669215861125849187374114990234375;-0.3636685669204331450288236737833358347415924072265625]
      mask Display: e = 0.06;c1 = [120 150 230]/255;c2 = ([120 150 230]+0)/383;c3 = ([120 150 230]+128)/383;patch([0 1 1 0],[0 0 1 1],c1);patch([0 1 1 1-e 1-e 0+e],[0 0 1 1-e 0+e 0+e],c2);patch([0 0 1 1-e 0+e 0+e],[0 1 1 1-e 1-e 0+e],c3);plot([0 1 1 0 0],[0 0 1 1 0]);disp('b');
  netsum : Sum  Inputs=2  InputSameDT=on  SaturateOnIntegerOverflow=on  OutDataTypeStr=Inherit: Same as first input
      mask Display: e = 0.06;c1 = [120 150 230]/255;c2 = ([120 150 230]+0)/383;c3 = ([120 150 230]+128)/383;patch([0 1 1 0],[0 0 1 1],c1);patch([0 1 1 1-e 1-e 0+e],[0 0 1 1-e 0+e 0+e],c2);patch([0 0 1 1-e 0+e 0+e],[0 1 1 1-e 1-e 0+e],c3);plot([0 1 1 0 0],[0 0 1 1 0]);disp('+');
  poslin : neural/Transfer Functions/poslin
      settings: SourceProductBaseCode=NN
  "a{2}" : Outport  InitialOutput=[0;0;0;0;0;0;0;0;0;0;0;0]
      mask Display: e = 0.06;c1 = [120 230 180]/255;c2 = ([120 230 180]+0)/(256+128);c3 = ([120 230 180]+128)/(256+128);patch([0 1 1 0],[0 0 1 1],c1);patch([0 1 1 1-e 1-e 0+e],[0 0 1 1-e 0+e 0+e],c2);patch([0 0 1 1-e 0+e 0+e],[0 1 1 1-e 1-e 0+e],c3);plot([0 1 1 0 0],[0 0 1 1 0]);
  wires:
  "a{1} "/1 -> Delays 1/1("p{2}")
  Delays 1/1("pd{2,1}") -> "LW{2,1}"/1("ad{2,1}")
  "LW{2,1}"/1("lz{2,1}") -> netsum/1
  "b{2}"/1 -> netsum/2
  netsum/1 -> poslin/1
  poslin/1 -> "a{2}"/1

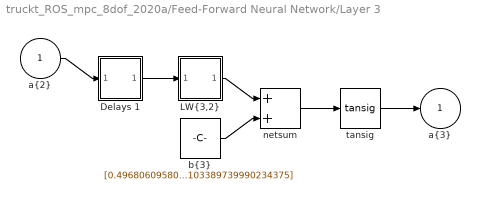
== system truckt_ROS_mpc_8dof_2020a/Feed-Forward Neural Network/Layer 3 ==
  "a{2} " : Inport  PortDimensions=12  SampleTime=0.0005
      mask Display: e = 0.06;c1 = [120 230 180]/255;c2 = ([120 230 180]+0)/(256+128);c3 = ([120 230 180]+128)/(256+128);patch([0 1 1 0],[0 0 1 1],c1);patch([0 1 1 1-e 1-e 0+e],[0 0 1 1-e 0+e 0+e],c2);patch([0 0 1 1-e 0+e 0+e],[0 1 1 1-e 1-e 0+e],c3);plot([0 1 1 0 0],[0 0 1 1 0]);
  Delays 1 : Subsystem
      mask Display: e = 0.06;c1 = [120 150 230]/255;c2 = ([120 150 230]+0)/383;c3 = ([120 150 230]+128)/383;patch([0 1 1 0],[0 0 1 1],c1);patch([0 1 1 1-e 1-e 0+e],[0 0 1 1-e 0+e 0+e],c2);patch([0 0 1 1-e 0+e 0+e],[0 1 1 1-e 1-e 0+e],c3);plot([0 1 1 0 0],[0 0 1 1 0]);disp('0');
  "LW{3,2}" : Subsystem
      mask Display: e = 0.06;c1 = [120 150 230]/255;c2 = ([120 150 230]+0)/383;c3 = ([120 150 230]+128)/383;patch([0 1 1 0],[0 0 1 1],c1);patch([0 1 1 1-e 1-e 0+e],[0 0 1 1-e 0+e 0+e],c2);patch([0 0 1 1-e 0+e 0+e],[0 1 1 1-e 1-e 0+e],c3);plot([0 1 1 0 0],[0 0 1 1 0]);disp('W');
  "b{3}" : Constant  Value=[0.496806095800611136059643513362971134483814239501953125;1.716998848888683593116866177297197282314300537109375;2.06273818817892706789507428766228258609771728515625;2.0468692729068234115175073384307324886322021484375;-0.01330929264457336204385828892782228649593889713287353515625;-0.877196684922304736886644604965113103389739990234375]
      mask Display: e = 0.06;c1 = [120 150 230]/255;c2 = ([120 150 230]+0)/383;c3 = ([120 150 230]+128)/383;patch([0 1 1 0],[0 0 1 1],c1);patch([0 1 1 1-e 1-e 0+e],[0 0 1 1-e 0+e 0+e],c2);patch([0 0 1 1-e 0+e 0+e],[0 1 1 1-e 1-e 0+e],c3);plot([0 1 1 0 0],[0 0 1 1 0]);disp('b');
  netsum : Sum  Inputs=2  InputSameDT=on  SaturateOnIntegerOverflow=on  OutDataTypeStr=Inherit: Same as first input
      mask Display: e = 0.06;c1 = [120 150 230]/255;c2 = ([120 150 230]+0)/383;c3 = ([120 150 230]+128)/383;patch([0 1 1 0],[0 0 1 1],c1);patch([0 1 1 1-e 1-e 0+e],[0 0 1 1-e 0+e 0+e],c2);patch([0 0 1 1-e 0+e 0+e],[0 1 1 1-e 1-e 0+e],c3);plot([0 1 1 0 0],[0 0 1 1 0]);disp('+');
  tansig : neural/Transfer Functions/tansig
  "a{3}" : Outport  InitialOutput=[0;0;0;0;0;0]
      mask Display: e = 0.06;c1 = [120 230 180]/255;c2 = ([120 230 180]+0)/(256+128);c3 = ([120 230 180]+128)/(256+128);patch([0 1 1 0],[0 0 1 1],c1);patch([0 1 1 1-e 1-e 0+e],[0 0 1 1-e 0+e 0+e],c2);patch([0 0 1 1-e 0+e 0+e],[0 1 1 1-e 1-e 0+e],c3);plot([0 1 1 0 0],[0 0 1 1 0]);
  wires:
  "a{2} "/1 -> Delays 1/1("p{3}")
  Delays 1/1("pd{3,2}") -> "LW{3,2}"/1("ad{3,2}")
  "LW{3,2}"/1("lz{3,2}") -> netsum/1
  "b{3}"/1 -> netsum/2
  netsum/1 -> tansig/1
  tansig/1 -> "a{3}"/1

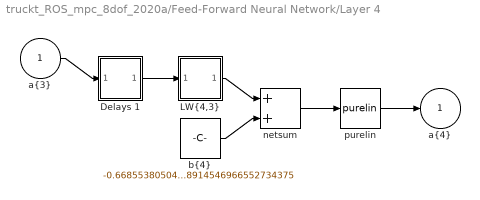
== system truckt_ROS_mpc_8dof_2020a/Feed-Forward Neural Network/Layer 4 ==
  "a{3} " : Inport  PortDimensions=6  SampleTime=0.0005
      mask Display: e = 0.06;c1 = [120 230 180]/255;c2 = ([120 230 180]+0)/(256+128);c3 = ([120 230 180]+128)/(256+128);patch([0 1 1 0],[0 0 1 1],c1);patch([0 1 1 1-e 1-e 0+e],[0 0 1 1-e 0+e 0+e],c2);patch([0 0 1 1-e 0+e 0+e],[0 1 1 1-e 1-e 0+e],c3);plot([0 1 1 0 0],[0 0 1 1 0]);
  Delays 1 : Subsystem
      mask Display: e = 0.06;c1 = [120 150 230]/255;c2 = ([120 150 230]+0)/383;c3 = ([120 150 230]+128)/383;patch([0 1 1 0],[0 0 1 1],c1);patch([0 1 1 1-e 1-e 0+e],[0 0 1 1-e 0+e 0+e],c2);patch([0 0 1 1-e 0+e 0+e],[0 1 1 1-e 1-e 0+e],c3);plot([0 1 1 0 0],[0 0 1 1 0]);disp('0');
  "LW{4,3}" : Subsystem
      mask Display: e = 0.06;c1 = [120 150 230]/255;c2 = ([120 150 230]+0)/383;c3 = ([120 150 230]+128)/383;patch([0 1 1 0],[0 0 1 1],c1);patch([0 1 1 1-e 1-e 0+e],[0 0 1 1-e 0+e 0+e],c2);patch([0 0 1 1-e 0+e 0+e],[0 1 1 1-e 1-e 0+e],c3);plot([0 1 1 0 0],[0 0 1 1 0]);disp('W');
  "b{4}" : Constant  Value=-0.66855380504418826514978491104557178914546966552734375
      mask Display: e = 0.06;c1 = [120 150 230]/255;c2 = ([120 150 230]+0)/383;c3 = ([120 150 230]+128)/383;patch([0 1 1 0],[0 0 1 1],c1);patch([0 1 1 1-e 1-e 0+e],[0 0 1 1-e 0+e 0+e],c2);patch([0 0 1 1-e 0+e 0+e],[0 1 1 1-e 1-e 0+e],c3);plot([0 1 1 0 0],[0 0 1 1 0]);disp('b');
  netsum : Sum  Inputs=2  InputSameDT=on  SaturateOnIntegerOverflow=on  OutDataTypeStr=Inherit: Same as first input
      mask Display: e = 0.06;c1 = [120 150 230]/255;c2 = ([120 150 230]+0)/383;c3 = ([120 150 230]+128)/383;patch([0 1 1 0],[0 0 1 1],c1);patch([0 1 1 1-e 1-e 0+e],[0 0 1 1-e 0+e 0+e],c2);patch([0 0 1 1-e 0+e 0+e],[0 1 1 1-e 1-e 0+e],c3);plot([0 1 1 0 0],[0 0 1 1 0]);disp('+');
  purelin : neural/Transfer Functions/purelin
  "a{4}" : Outport  InitialOutput=0
      mask Display: e = 0.06;c1 = [120 230 180]/255;c2 = ([120 230 180]+0)/(256+128);c3 = ([120 230 180]+128)/(256+128);patch([0 1 1 0],[0 0 1 1],c1);patch([0 1 1 1-e 1-e 0+e],[0 0 1 1-e 0+e 0+e],c2);patch([0 0 1 1-e 0+e 0+e],[0 1 1 1-e 1-e 0+e],c3);plot([0 1 1 0 0],[0 0 1 1 0]);
  wires:
  "a{3} "/1 -> Delays 1/1("p{4}")
  Delays 1/1("pd{4,3}") -> "LW{4,3}"/1("ad{4,3}")
  "LW{4,3}"/1("lz{4,3}") -> netsum/1
  "b{4}"/1 -> netsum/2
  netsum/1 -> purelin/1
  purelin/1 -> "a{4}"/1

== system truckt_ROS_mpc_8dof_2020a/Feed-Forward Neural Network/Process Input 1 ==
  x : Inport  PortDimensions=3  SampleTime=0.0005
      mask Display: e = 0.06;c1 = [120 230 180]/255;c2 = ([120 230 180]+0)/(256+128);c3 = ([120 230 180]+128)/(256+128);patch([0 1 1 0],[0 0 1 1],c1);patch([0 1 1 1-e 1-e 0+e],[0 0 1 1-e 0+e 0+e],c2);patch([0 0 1 1-e 0+e 0+e],[0 1 1 1-e 1-e 0+e],c3);plot([0 1 1 0 0],[0 0 1 1 0]);
  mapminmax : neural/Processing Functions/mapminmax  xmin=[-6.36999999999999655386773156351;-74.2088783047049673768924549222;0.00100000000000000002081668171172]  xmax=[11.0700000000000038369307731045;-29.9816675178919815891731559532;6.5240000000000000213162820728]  ymin=-1  ymax=1
  p : Outport  PortDimensions=3  SampleTime=0.0005
      mask Display: e = 0.06;c1 = [120 230 180]/255;c2 = ([120 230 180]+0)/(256+128);c3 = ([120 230 180]+128)/(256+128);patch([0 1 1 0],[0 0 1 1],c1);patch([0 1 1 1-e 1-e 0+e],[0 0 1 1-e 0+e 0+e],c2);patch([0 0 1 1-e 0+e 0+e],[0 1 1 1-e 1-e 0+e],c3);plot([0 1 1 0 0],[0 0 1 1 0]);
  wires:
  x/1 -> mapminmax/1
  mapminmax/1 -> p/1

== system truckt_ROS_mpc_8dof_2020a/Feed-Forward Neural Network/Process Output 1 ==
  a : Inport  PortDimensions=1  SampleTime=0.0005
      mask Display: e = 0.06;c1 = [120 230 180]/255;c2 = ([120 230 180]+0)/(256+128);c3 = ([120 230 180]+128)/(256+128);patch([0 1 1 0],[0 0 1 1],c1);patch([0 1 1 1-e 1-e 0+e],[0 0 1 1-e 0+e 0+e],c2);patch([0 0 1 1-e 0+e 0+e],[0 1 1 1-e 1-e 0+e],c3);plot([0 1 1 0 0],[0 0 1 1 0]);
  mapminmax_reverse : neural/Processing Functions/mapminmax_reverse  xmin=-3.05443652937453746787355157721  xmax=4.00459973833020210776112435269  ymin=-1  ymax=1
  y : Outport  PortDimensions=1  SampleTime=0.0005
      mask Display: e = 0.06;c1 = [120 230 180]/255;c2 = ([120 230 180]+0)/(256+128);c3 = ([120 230 180]+128)/(256+128);patch([0 1 1 0],[0 0 1 1],c1);patch([0 1 1 1-e 1-e 0+e],[0 0 1 1-e 0+e 0+e],c2);patch([0 0 1 1-e 0+e 0+e],[0 1 1 1-e 1-e 0+e],c3);plot([0 1 1 0 0],[0 0 1 1 0]);
  wires:
  a/1 -> mapminmax_reverse/1
  mapminmax_reverse/1 -> y/1

== system truckt_ROS_mpc_8dof_2020a/Feed-Forward Neural Network/Layer 1/Delays 1 ==
  "p{1}" : Inport  PortDimensions=3  SampleTime=0.0005
      mask Display: e = 0.06;c1 = [120 230 180]/255;c2 = ([120 230 180]+0)/(256+128);c3 = ([120 230 180]+128)/(256+128);patch([0 1 1 0],[0 0 1 1],c1);patch([0 1 1 1-e 1-e 0+e],[0 0 1 1-e 0+e 0+e],c2);patch([0 0 1 1-e 0+e 0+e],[0 1 1 1-e 1-e 0+e],c3);plot([0 1 1 0 0],[0 0 1 1 0]);
  mux : Mux  Inputs=1
      mask Display: e = 0.06;c1 = [120 150 230]/255;c2 = ([120 150 230]+0)/383;c3 = ([120 150 230]+128)/383;patch([0 1 1 0],[0 0 1 1],c1);patch([0 1 1 1-e 1-e 0+e],[0 0 1 1-e 0+e 0+e],c2);patch([0 0 1 1-e 0+e 0+e],[0 1 1 1-e 1-e 0+e],c3);plot([0 1 1 0 0],[0 0 1 1 0]);disp('Mux')
  "pd{1,1}" : Outport
      mask Display: e = 0.06;c1 = [120 230 180]/255;c2 = ([120 230 180]+0)/(256+128);c3 = ([120 230 180]+128)/(256+128);patch([0 1 1 0],[0 0 1 1],c1);patch([0 1 1 1-e 1-e 0+e],[0 0 1 1-e 0+e 0+e],c2);patch([0 0 1 1-e 0+e 0+e],[0 1 1 1-e 1-e 0+e],c3);plot([0 1 1 0 0],[0 0 1 1 0]);
  wires:
  "p{1}"/1 -> mux/1
  mux/1 -> "pd{1,1}"/1

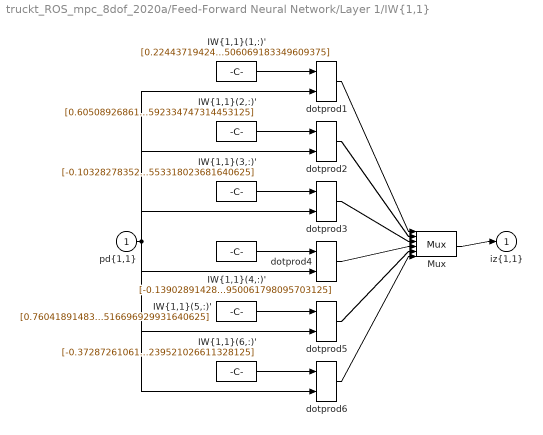
== system truckt_ROS_mpc_8dof_2020a/Feed-Forward Neural Network/Layer 1/IW{1,1} ==
  "pd{1,1}" : Inport  PortDimensions=3  SampleTime=0.0005
      mask Display: e = 0.06;c1 = [120 230 180]/255;c2 = ([120 230 180]+0)/(256+128);c3 = ([120 230 180]+128)/(256+128);patch([0 1 1 0],[0 0 1 1],c1);patch([0 1 1 1-e 1-e 0+e],[0 0 1 1-e 0+e 0+e],c2);patch([0 0 1 1-e 0+e 0+e],[0 1 1 1-e 1-e 0+e],c3);plot([0 1 1 0 0],[0 0 1 1 0]);
  "IW{1,1}(1,:)'" : Constant  Value=[0.224437194248272409158317941546556539833545684814453125;-0.63298872538204353777047117546317167580127716064453125;-0.6852859746264987617081487769610248506069183349609375]
      mask Display: e = 0.06;c1 = [120 150 230]/255;c2 = ([120 150 230]+0)/383;c3 = ([120 150 230]+128)/383;patch([0 1 1 0],[0 0 1 1],c1);patch([0 1 1 1-e 1-e 0+e],[0 0 1 1-e 0+e 0+e],c2);patch([0 0 1 1-e 0+e 0+e],[0 1 1 1-e 1-e 0+e],c3);plot([0 1 1 0 0],[0 0 1 1 0]);disp('Weights');
  "IW{1,1}(2,:)'" : Constant  Value=[0.6050892686156268407415836918517015874385833740234375;-0.316879128175024005198423537876806221902370452880859375;0.044744899328895304524422726899501867592334747314453125]
      mask Display: e = 0.06;c1 = [120 150 230]/255;c2 = ([120 150 230]+0)/383;c3 = ([120 150 230]+128)/383;patch([0 1 1 0],[0 0 1 1],c1);patch([0 1 1 1-e 1-e 0+e],[0 0 1 1-e 0+e 0+e],c2);patch([0 0 1 1-e 0+e 0+e],[0 1 1 1-e 1-e 0+e],c3);plot([0 1 1 0 0],[0 0 1 1 0]);disp('Weights');
  "IW{1,1}(3,:)'" : Constant  Value=[-0.103282783528666988193123188466415740549564361572265625;-0.240764573286563809961791093883221037685871124267578125;0.89017105450226952090275744922109879553318023681640625]
      mask Display: e = 0.06;c1 = [120 150 230]/255;c2 = ([120 150 230]+0)/383;c3 = ([120 150 230]+128)/383;patch([0 1 1 0],[0 0 1 1],c1);patch([0 1 1 1-e 1-e 0+e],[0 0 1 1-e 0+e 0+e],c2);patch([0 0 1 1-e 0+e 0+e],[0 1 1 1-e 1-e 0+e],c3);plot([0 1 1 0 0],[0 0 1 1 0]);disp('Weights');
  "IW{1,1}(4,:)'" : Constant  Value=[-0.1390289142860972881887704488690360449254512786865234375;0.34119606768922616790717938783927820622920989990234375;0.82894492406411413032429891245556063950061798095703125]
      mask Display: e = 0.06;c1 = [120 150 230]/255;c2 = ([120 150 230]+0)/383;c3 = ([120 150 230]+128)/383;patch([0 1 1 0],[0 0 1 1],c1);patch([0 1 1 1-e 1-e 0+e],[0 0 1 1-e 0+e 0+e],c2);patch([0 0 1 1-e 0+e 0+e],[0 1 1 1-e 1-e 0+e],c3);plot([0 1 1 0 0],[0 0 1 1 0]);disp('Weights');
  "IW{1,1}(5,:)'" : Constant  Value=[0.76041891483327506140454943306394852697849273681640625;-0.331878455308418141012083424357115291059017181396484375;0.429452455542128463950035666130133904516696929931640625]
      mask Display: e = 0.06;c1 = [120 150 230]/255;c2 = ([120 150 230]+0)/383;c3 = ([120 150 230]+128)/383;patch([0 1 1 0],[0 0 1 1],c1);patch([0 1 1 1-e 1-e 0+e],[0 0 1 1-e 0+e 0+e],c2);patch([0 0 1 1-e 0+e 0+e],[0 1 1 1-e 1-e 0+e],c3);plot([0 1 1 0 0],[0 0 1 1 0]);disp('Weights');
  "IW{1,1}(6,:)'" : Constant  Value=[-0.372872610611773069866359264779021032154560089111328125;-0.55848278055298117283911096819792874157428741455078125;-0.485208932450945429337707537342794239521026611328125]
      mask Display: e = 0.06;c1 = [120 150 230]/255;c2 = ([120 150 230]+0)/383;c3 = ([120 150 230]+128)/383;patch([0 1 1 0],[0 0 1 1],c1);patch([0 1 1 1-e 1-e 0+e],[0 0 1 1-e 0+e 0+e],c2);patch([0 0 1 1-e 0+e 0+e],[0 1 1 1-e 1-e 0+e],c3);plot([0 1 1 0 0],[0 0 1 1 0]);disp('Weights');
  Mux : Mux  Inputs=6
      mask Display: e = 0.06;c1 = [120 150 230]/255;c2 = ([120 150 230]+0)/383;c3 = ([120 150 230]+128)/383;patch([0 1 1 0],[0 0 1 1],c1);patch([0 1 1 1-e 1-e 0+e],[0 0 1 1-e 0+e 0+e],c2);patch([0 0 1 1-e 0+e 0+e],[0 1 1 1-e 1-e 0+e],c3);plot([0 1 1 0 0],[0 0 1 1 0]);disp('Mux');
  dotprod{1..6} (6 alike) : neural/Weight Functions/dotprod
  "iz{1,1}" : Outport
      mask Display: e = 0.06;c1 = [120 230 180]/255;c2 = ([120 230 180]+0)/(256+128);c3 = ([120 230 180]+128)/(256+128);patch([0 1 1 0],[0 0 1 1],c1);patch([0 1 1 1-e 1-e 0+e],[0 0 1 1-e 0+e 0+e],c2);patch([0 0 1 1-e 0+e 0+e],[0 1 1 1-e 1-e 0+e],c3);plot([0 1 1 0 0],[0 0 1 1 0]);
  wires:
  "IW{1,1}(1,:)'"/1 -> dotprod1/1
  "pd{1,1}"/1 -> dotprod1/2, dotprod2/2, dotprod3/2, dotprod4/2, dotprod5/2, dotprod6/2
  dotprod1/1 -> Mux/1
  "IW{1,1}(2,:)'"/1 -> dotprod2/1
  dotprod2/1 -> Mux/2
  "IW{1,1}(3,:)'"/1 -> dotprod3/1
  dotprod3/1 -> Mux/3
  "IW{1,1}(4,:)'"/1 -> dotprod4/1
  dotprod4/1 -> Mux/4
  "IW{1,1}(5,:)'"/1 -> dotprod5/1
  dotprod5/1 -> Mux/5
  "IW{1,1}(6,:)'"/1 -> dotprod6/1
  dotprod6/1 -> Mux/6
  Mux/1 -> "iz{1,1}"/1

== system truckt_ROS_mpc_8dof_2020a/Feed-Forward Neural Network/Layer 2/Delays 1 ==
  "p{2}" : Inport  PortDimensions=6  SampleTime=0.0005
      mask Display: e = 0.06;c1 = [120 230 180]/255;c2 = ([120 230 180]+0)/(256+128);c3 = ([120 230 180]+128)/(256+128);patch([0 1 1 0],[0 0 1 1],c1);patch([0 1 1 1-e 1-e 0+e],[0 0 1 1-e 0+e 0+e],c2);patch([0 0 1 1-e 0+e 0+e],[0 1 1 1-e 1-e 0+e],c3);plot([0 1 1 0 0],[0 0 1 1 0]);
  mux : Mux  Inputs=1
      mask Display: e = 0.06;c1 = [120 150 230]/255;c2 = ([120 150 230]+0)/383;c3 = ([120 150 230]+128)/383;patch([0 1 1 0],[0 0 1 1],c1);patch([0 1 1 1-e 1-e 0+e],[0 0 1 1-e 0+e 0+e],c2);patch([0 0 1 1-e 0+e 0+e],[0 1 1 1-e 1-e 0+e],c3);plot([0 1 1 0 0],[0 0 1 1 0]);disp('Mux')
  "pd{2,1}" : Outport
      mask Display: e = 0.06;c1 = [120 230 180]/255;c2 = ([120 230 180]+0)/(256+128);c3 = ([120 230 180]+128)/(256+128);patch([0 1 1 0],[0 0 1 1],c1);patch([0 1 1 1-e 1-e 0+e],[0 0 1 1-e 0+e 0+e],c2);patch([0 0 1 1-e 0+e 0+e],[0 1 1 1-e 1-e 0+e],c3);plot([0 1 1 0 0],[0 0 1 1 0]);
  wires:
  "p{2}"/1 -> mux/1
  mux/1 -> "pd{2,1}"/1

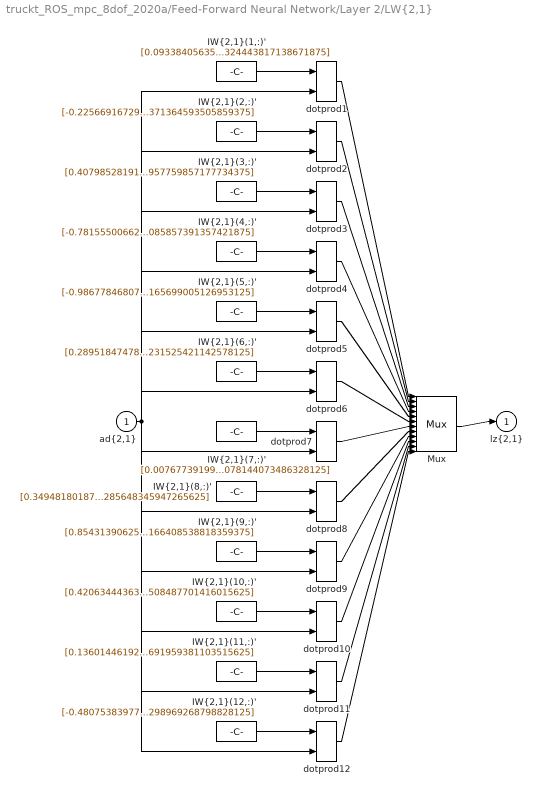
== system truckt_ROS_mpc_8dof_2020a/Feed-Forward Neural Network/Layer 2/LW{2,1} ==
  "ad{2,1}" : Inport  PortDimensions=6  SampleTime=0.0005
      mask Display: e = 0.06;c1 = [120 230 180]/255;c2 = ([120 230 180]+0)/(256+128);c3 = ([120 230 180]+128)/(256+128);patch([0 1 1 0],[0 0 1 1],c1);patch([0 1 1 1-e 1-e 0+e],[0 0 1 1-e 0+e 0+e],c2);patch([0 0 1 1-e 0+e 0+e],[0 1 1 1-e 1-e 0+e],c3);plot([0 1 1 0 0],[0 0 1 1 0]);
  "IW{2,1}(1,:)'" : Constant  Value=[0.0933840563570031978457564036943949759006500244140625;-0.6941715198521276608545349517953582108020782470703125;0.7564998596566898658721811443683691322803497314453125;0.5565420599909083332335058003081940114498138427734375;0.217771077394351753042656127945519983768463134765625;-0.17229988011105745737694405761430971324443817138671875]
      mask Display: e = 0.06;c1 = [120 150 230]/255;c2 = ([120 150 230]+0)/383;c3 = ([120 150 230]+128)/383;patch([0 1 1 0],[0 0 1 1],c1);patch([0 1 1 1-e 1-e 0+e],[0 0 1 1-e 0+e 0+e],c2);patch([0 0 1 1-e 0+e 0+e],[0 1 1 1-e 1-e 0+e],c3);plot([0 1 1 0 0],[0 0 1 1 0]);disp('weights');
  "IW{2,1}(10,:)'" : Constant  Value=[0.420634443631284771214495776803232729434967041015625;0.919079656801795152887279982678592205047607421875;0.38899722104157985480554771129391156136989593505859375;-0.77063601104271983732729722760268487036228179931640625;-0.450822666829107043806601495816721580922603607177734375;0.7097421980723110923605645439238287508487701416015625]
      mask Display: e = 0.06;c1 = [120 150 230]/255;c2 = ([120 150 230]+0)/383;c3 = ([120 150 230]+128)/383;patch([0 1 1 0],[0 0 1 1],c1);patch([0 1 1 1-e 1-e 0+e],[0 0 1 1-e 0+e 0+e],c2);patch([0 0 1 1-e 0+e 0+e],[0 1 1 1-e 1-e 0+e],c3);plot([0 1 1 0 0],[0 0 1 1 0]);disp('weights');
  "IW{2,1}(11,:)'" : Constant  Value=[0.136014461927510321714862584485672414302825927734375;0.78258184957946019810748339295969344675540924072265625;-0.1867160575215238427215780347978579811751842498779296875;0.8369279027338001331060013399110175669193267822265625;0.410424118903048140705180912846117280423641204833984375;-0.351712888103358933822306653382838703691959381103515625]
      mask Display: e = 0.06;c1 = [120 150 230]/255;c2 = ([120 150 230]+0)/383;c3 = ([120 150 230]+128)/383;patch([0 1 1 0],[0 0 1 1],c1);patch([0 1 1 1-e 1-e 0+e],[0 0 1 1-e 0+e 0+e],c2);patch([0 0 1 1-e 0+e 0+e],[0 1 1 1-e 1-e 0+e],c3);plot([0 1 1 0 0],[0 0 1 1 0]);disp('weights');
  "IW{2,1}(12,:)'" : Constant  Value=[-0.480753839779001879151110188104212284088134765625;-0.639063780622896704386448618606664240360260009765625;-0.3516070730659208720680908299982547760009765625;0.941045573912211441580666360096074640750885009765625;0.5803458700486687771302740657120011746883392333984375;-0.210685116872369793128427772899158298969268798828125]
      mask Display: e = 0.06;c1 = [120 150 230]/255;c2 = ([120 150 230]+0)/383;c3 = ([120 150 230]+128)/383;patch([0 1 1 0],[0 0 1 1],c1);patch([0 1 1 1-e 1-e 0+e],[0 0 1 1-e 0+e 0+e],c2);patch([0 0 1 1-e 0+e 0+e],[0 1 1 1-e 1-e 0+e],c3);plot([0 1 1 0 0],[0 0 1 1 0]);disp('weights');
  "IW{2,1}(2,:)'" : Constant  Value=[-0.22566916729820551967833353046444244682788848876953125;0.74750481879836760956692387480870820581912994384765625;-1.150766244719649389338655964820645749568939208984375;-0.03226190050673928555458047640058794058859348297119140625;0.445411271681787346299330465626553632318973541259765625;-1.04490691323366657883298103115521371364593505859375]
      mask Display: e = 0.06;c1 = [120 150 230]/255;c2 = ([120 150 230]+0)/383;c3 = ([120 150 230]+128)/383;patch([0 1 1 0],[0 0 1 1],c1);patch([0 1 1 1-e 1-e 0+e],[0 0 1 1-e 0+e 0+e],c2);patch([0 0 1 1-e 0+e 0+e],[0 1 1 1-e 1-e 0+e],c3);plot([0 1 1 0 0],[0 0 1 1 0]);disp('weights');
  "IW{2,1}(3,:)'" : Constant  Value=[0.40798528191055838387768517350195907056331634521484375;-0.7293259653551207311039661362883634865283966064453125;-0.56290434577644699043474929567310027778148651123046875;-0.740877192382068727738442248664796352386474609375;-0.3944953485404363302535557522787712514400482177734375;-0.72264491935812935619054542257799766957759857177734375]
      mask Display: e = 0.06;c1 = [120 150 230]/255;c2 = ([120 150 230]+0)/383;c3 = ([120 150 230]+128)/383;patch([0 1 1 0],[0 0 1 1],c1);patch([0 1 1 1-e 1-e 0+e],[0 0 1 1-e 0+e 0+e],c2);patch([0 0 1 1-e 0+e 0+e],[0 1 1 1-e 1-e 0+e],c3);plot([0 1 1 0 0],[0 0 1 1 0]);disp('weights');
  "IW{2,1}(4,:)'" : Constant  Value=[-0.7815550066226901737564958239090628921985626220703125;-0.43920598862091342340363553375937044620513916015625;-0.9822899398027995498949849206837825477123260498046875;-0.2392728811746656081282935701892711222171783447265625;-0.0819552118429618392525526360259391367435455322265625;0.2750452786799950644081036443822085857391357421875]
      mask Display: e = 0.06;c1 = [120 150 230]/255;c2 = ([120 150 230]+0)/383;c3 = ([120 150 230]+128)/383;patch([0 1 1 0],[0 0 1 1],c1);patch([0 1 1 1-e 1-e 0+e],[0 0 1 1-e 0+e 0+e],c2);patch([0 0 1 1-e 0+e 0+e],[0 1 1 1-e 1-e 0+e],c3);plot([0 1 1 0 0],[0 0 1 1 0]);disp('weights');
  "IW{2,1}(5,:)'" : Constant  Value=[-0.986778468071595415977981247124262154102325439453125;-0.48114510404508070706697253626771271228790283203125;0.3431870686257465496993290798855014145374298095703125;-0.2068615095779164914091552418540231883525848388671875;-0.9039427736352718678602968793711625039577484130859375;-0.1514288375658001672974251050618477165699005126953125]
      mask Display: e = 0.06;c1 = [120 150 230]/255;c2 = ([120 150 230]+0)/383;c3 = ([120 150 230]+128)/383;patch([0 1 1 0],[0 0 1 1],c1);patch([0 1 1 1-e 1-e 0+e],[0 0 1 1-e 0+e 0+e],c2);patch([0 0 1 1-e 0+e 0+e],[0 1 1 1-e 1-e 0+e],c3);plot([0 1 1 0 0],[0 0 1 1 0]);disp('weights');
  "IW{2,1}(6,:)'" : Constant  Value=[0.289518474781735812850769207216217182576656341552734375;0.49624645331644956502969989742268808186054229736328125;0.7306319806818504236645139826578088104724884033203125;0.2041848038870807402478391168187954463064670562744140625;-0.26733131924891340158723096465109847486019134521484375;-0.05739387591178930769775234921326045878231525421142578125]
      mask Display: e = 0.06;c1 = [120 150 230]/255;c2 = ([120 150 230]+0)/383;c3 = ([120 150 230]+128)/383;patch([0 1 1 0],[0 0 1 1],c1);patch([0 1 1 1-e 1-e 0+e],[0 0 1 1-e 0+e 0+e],c2);patch([0 0 1 1-e 0+e 0+e],[0 1 1 1-e 1-e 0+e],c3);plot([0 1 1 0 0],[0 0 1 1 0]);disp('weights');
  "IW{2,1}(7,:)'" : Constant  Value=[0.007677391993178008140763513011961549636907875537872314453125;0.450847943611103529892858432503999210894107818603515625;-0.2626504537842055952978626010008156299591064453125;-0.83327208469632318976749729699804447591304779052734375;-0.3004006108321359835855446362984366714954376220703125;-0.50382483197474414726713121126522310078144073486328125]
      mask Display: e = 0.06;c1 = [120 150 230]/255;c2 = ([120 150 230]+0)/383;c3 = ([120 150 230]+128)/383;patch([0 1 1 0],[0 0 1 1],c1);patch([0 1 1 1-e 1-e 0+e],[0 0 1 1-e 0+e 0+e],c2);patch([0 0 1 1-e 0+e 0+e],[0 1 1 1-e 1-e 0+e],c3);plot([0 1 1 0 0],[0 0 1 1 0]);disp('weights');
  "IW{2,1}(8,:)'" : Constant  Value=[0.349481801874595710000193093947018496692180633544921875;0.50233657626711536448027572987484745681285858154296875;-0.2395554425237038653762056128471158444881439208984375;0.065115835084826712009231641786755062639713287353515625;-0.63503147990537212042028158975881524384021759033203125;-0.5628767585490754843391414397046901285648345947265625]
      mask Display: e = 0.06;c1 = [120 150 230]/255;c2 = ([120 150 230]+0)/383;c3 = ([120 150 230]+128)/383;patch([0 1 1 0],[0 0 1 1],c1);patch([0 1 1 1-e 1-e 0+e],[0 0 1 1-e 0+e 0+e],c2);patch([0 0 1 1-e 0+e 0+e],[0 1 1 1-e 1-e 0+e],c3);plot([0 1 1 0 0],[0 0 1 1 0]);disp('weights');
  "IW{2,1}(9,:)'" : Constant  Value=[0.85431390625108416525534948959830217063426971435546875;0.463870938360337492500917733195819891989231109619140625;-0.41330276989663550235576394698000513017177581787109375;0.89237210875835126788757634130888618528842926025390625;0.70638344501733574265500692490604706108570098876953125;0.63707020519249224488333993576816283166408538818359375]
      mask Display: e = 0.06;c1 = [120 150 230]/255;c2 = ([120 150 230]+0)/383;c3 = ([120 150 230]+128)/383;patch([0 1 1 0],[0 0 1 1],c1);patch([0 1 1 1-e 1-e 0+e],[0 0 1 1-e 0+e 0+e],c2);patch([0 0 1 1-e 0+e 0+e],[0 1 1 1-e 1-e 0+e],c3);plot([0 1 1 0 0],[0 0 1 1 0]);disp('weights');
  Mux : Mux  Inputs=12
      mask Display: e = 0.06;c1 = [120 150 230]/255;c2 = ([120 150 230]+0)/383;c3 = ([120 150 230]+128)/383;patch([0 1 1 0],[0 0 1 1],c1);patch([0 1 1 1-e 1-e 0+e],[0 0 1 1-e 0+e 0+e],c2);patch([0 0 1 1-e 0+e 0+e],[0 1 1 1-e 1-e 0+e],c3);plot([0 1 1 0 0],[0 0 1 1 0]);disp('Mux');
  dotprod{1..12} (12 alike) : neural/Weight Functions/dotprod
  "lz{2,1}" : Outport
      mask Display: e = 0.06;c1 = [120 230 180]/255;c2 = ([120 230 180]+0)/(256+128);c3 = ([120 230 180]+128)/(256+128);patch([0 1 1 0],[0 0 1 1],c1);patch([0 1 1 1-e 1-e 0+e],[0 0 1 1-e 0+e 0+e],c2);patch([0 0 1 1-e 0+e 0+e],[0 1 1 1-e 1-e 0+e],c3);plot([0 1 1 0 0],[0 0 1 1 0]);
  wires:
  "IW{2,1}(1,:)'"/1 -> dotprod1/1
  "ad{2,1}"/1 -> dotprod1/2, dotprod2/2, dotprod3/2, dotprod4/2, dotprod5/2, dotprod6/2, dotprod7/2, dotprod8/2, dotprod9/2, dotprod10/2, dotprod11/2, dotprod12/2
  dotprod1/1 -> Mux/1
  "IW{2,1}(2,:)'"/1 -> dotprod2/1
  dotprod2/1 -> Mux/2
  "IW{2,1}(3,:)'"/1 -> dotprod3/1
  dotprod3/1 -> Mux/3
  "IW{2,1}(4,:)'"/1 -> dotprod4/1
  dotprod4/1 -> Mux/4
  "IW{2,1}(5,:)'"/1 -> dotprod5/1
  dotprod5/1 -> Mux/5
  "IW{2,1}(6,:)'"/1 -> dotprod6/1
  dotprod6/1 -> Mux/6
  "IW{2,1}(7,:)'"/1 -> dotprod7/1
  dotprod7/1 -> Mux/7
  "IW{2,1}(8,:)'"/1 -> dotprod8/1
  dotprod8/1 -> Mux/8
  "IW{2,1}(9,:)'"/1 -> dotprod9/1
  dotprod9/1 -> Mux/9
  "IW{2,1}(10,:)'"/1 -> dotprod10/1
  dotprod10/1 -> Mux/10
  "IW{2,1}(11,:)'"/1 -> dotprod11/1
  dotprod11/1 -> Mux/11
  "IW{2,1}(12,:)'"/1 -> dotprod12/1
  dotprod12/1 -> Mux/12
  Mux/1 -> "lz{2,1}"/1

== system truckt_ROS_mpc_8dof_2020a/Feed-Forward Neural Network/Layer 3/Delays 1 ==
  "p{3}" : Inport  PortDimensions=12  SampleTime=0.0005
      mask Display: e = 0.06;c1 = [120 230 180]/255;c2 = ([120 230 180]+0)/(256+128);c3 = ([120 230 180]+128)/(256+128);patch([0 1 1 0],[0 0 1 1],c1);patch([0 1 1 1-e 1-e 0+e],[0 0 1 1-e 0+e 0+e],c2);patch([0 0 1 1-e 0+e 0+e],[0 1 1 1-e 1-e 0+e],c3);plot([0 1 1 0 0],[0 0 1 1 0]);
  mux : Mux  Inputs=1
      mask Display: e = 0.06;c1 = [120 150 230]/255;c2 = ([120 150 230]+0)/383;c3 = ([120 150 230]+128)/383;patch([0 1 1 0],[0 0 1 1],c1);patch([0 1 1 1-e 1-e 0+e],[0 0 1 1-e 0+e 0+e],c2);patch([0 0 1 1-e 0+e 0+e],[0 1 1 1-e 1-e 0+e],c3);plot([0 1 1 0 0],[0 0 1 1 0]);disp('Mux')
  "pd{3,2}" : Outport
      mask Display: e = 0.06;c1 = [120 230 180]/255;c2 = ([120 230 180]+0)/(256+128);c3 = ([120 230 180]+128)/(256+128);patch([0 1 1 0],[0 0 1 1],c1);patch([0 1 1 1-e 1-e 0+e],[0 0 1 1-e 0+e 0+e],c2);patch([0 0 1 1-e 0+e 0+e],[0 1 1 1-e 1-e 0+e],c3);plot([0 1 1 0 0],[0 0 1 1 0]);
  wires:
  "p{3}"/1 -> mux/1
  mux/1 -> "pd{3,2}"/1
